simulink library "Lib_FileLoggerMultipacket"  (R2012b)
settings: Solver=ode45  StartTime=0.0  StopTime=10.0  RelTol=1e-3
undefined symbols (not defined in the file): macaddr, modelConstants
libraries: Lib_FileLoggerMultipacket x5, simulink x3, xpcutilitieslib x1, dspswit3 x1, dspmtrx3 x1, libBusSerialize x1
settings Model: Creator=gilja  LastModifiedBy=Chethan

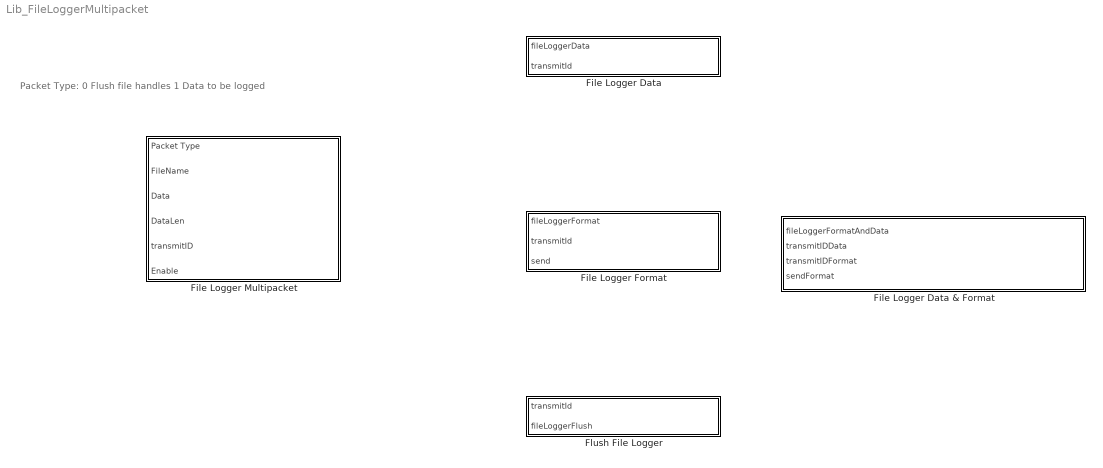
== system Lib_FileLoggerMultipacket ==
  note: Packet Type:
      | 0 Flush file handles
      | 1 Data to be logged
  File Logger Data : Subsystem
  File Logger Data & Format : Subsystem
  File Logger Format : Subsystem
  File Logger Multipacket : Subsystem
  Flush File Logger : Subsystem

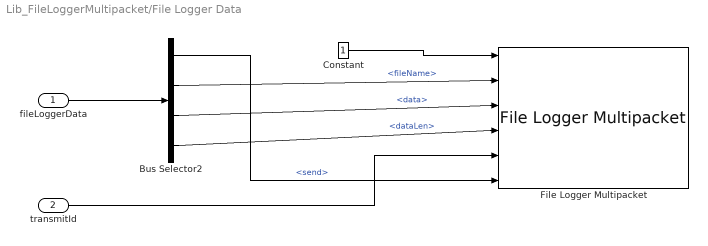
== system Lib_FileLoggerMultipacket/File Logger Data ==
  fileLoggerData : Inport  OutDataTypeStr=Bus: fileLoggerData
  transmitId : Inport  Port=2  OutDataTypeStr=uint8
  Bus Selector2 : BusSelector  OutputSignals=send,fileName,data,dataLen
  Constant : Constant  OutDataTypeStr=boolean
  File Logger Multipacket : Lib_FileLoggerMultipacket/File Logger Multipacket
  wires:
  fileLoggerData/1 -> Bus Selector2/1
  Constant/1 -> File Logger Multipacket/1
  Bus Selector2/1 -> File Logger Multipacket/6  "<send>"
  Bus Selector2/4 -> File Logger Multipacket/4  "<dataLen>"
  Bus Selector2/3 -> File Logger Multipacket/3  "<data>"
  Bus Selector2/2 -> File Logger Multipacket/2  "<fileName>"
  transmitId/1 -> File Logger Multipacket/5

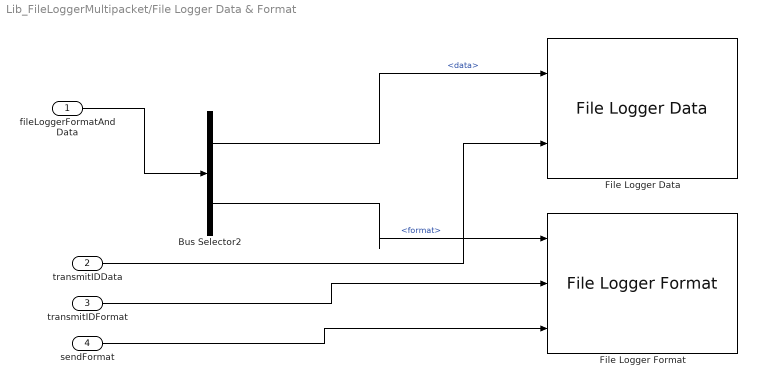
== system Lib_FileLoggerMultipacket/File Logger Data & Format ==
  fileLoggerFormatAndData : Inport  OutDataTypeStr=Bus: fileLoggerFormatAndData
  transmitIDData : Inport  Port=2  OutDataTypeStr=uint8
  transmitIDFormat : Inport  Port=3  OutDataTypeStr=uint8
  sendFormat : Inport  Port=4  OutDataTypeStr=boolean
  Bus Selector2 : BusSelector  OutputSignals=data,format
  File Logger Data : Lib_FileLoggerMultipacket/File Logger Data
  File Logger Format : Lib_FileLoggerMultipacket/File Logger Format
  wires:
  fileLoggerFormatAndData/1 -> Bus Selector2/1
  Bus Selector2/1 -> File Logger Data/1  "<data>"
  Bus Selector2/2 -> File Logger Format/1  "<format>"
  sendFormat/1 -> File Logger Format/3
  transmitIDData/1 -> File Logger Data/2
  transmitIDFormat/1 -> File Logger Format/2

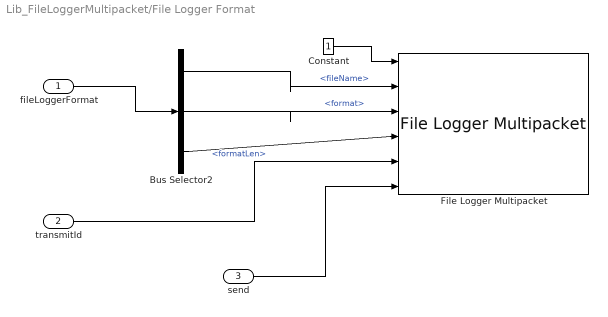
== system Lib_FileLoggerMultipacket/File Logger Format ==
  fileLoggerFormat : Inport  OutDataTypeStr=Bus: fileLoggerFormat
  transmitId : Inport  Port=2  OutDataTypeStr=uint8
  send : Inport  Port=3  OutDataTypeStr=boolean
  Bus Selector2 : BusSelector  OutputSignals=fileName,format,formatLen
  Constant : Constant  OutDataTypeStr=boolean
  File Logger Multipacket : Lib_FileLoggerMultipacket/File Logger Multipacket
  wires:
  fileLoggerFormat/1 -> Bus Selector2/1
  Constant/1 -> File Logger Multipacket/1
  Bus Selector2/3 -> File Logger Multipacket/4  "<formatLen>"
  Bus Selector2/2 -> File Logger Multipacket/3  "<format>"
  Bus Selector2/1 -> File Logger Multipacket/2  "<fileName>"
  send/1 -> File Logger Multipacket/6
  transmitId/1 -> File Logger Multipacket/5

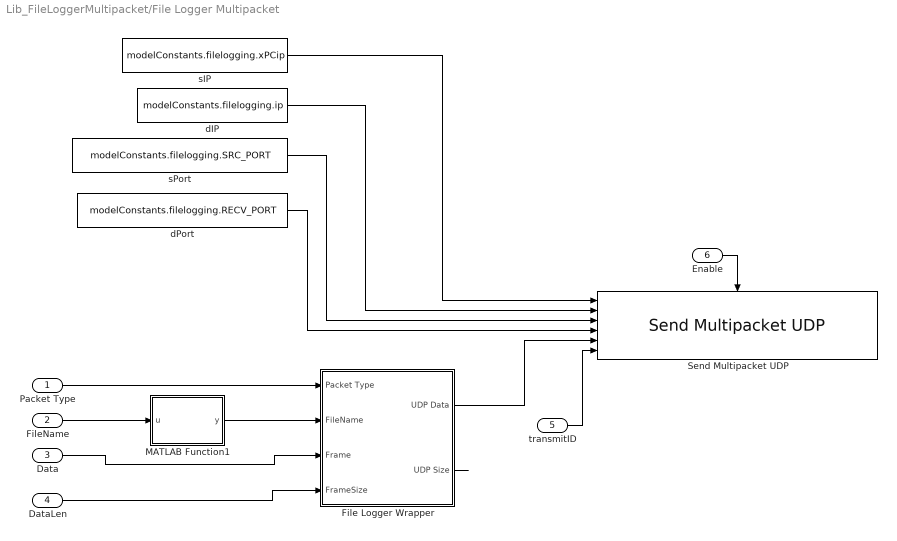
== system Lib_FileLoggerMultipacket/File Logger Multipacket ==
  Packet Type : Inport
  FileName : Inport  Port=2
  Data : Inport  Port=3
  DataLen : Inport  Port=4
  transmitID : Inport  Port=5
  Enable : Inport  Port=6
  File Logger Wrapper : Subsystem
  MATLAB Function1 : MATLAB Function  TreatAsAtomicUnit=on
  Send Multipacket UDP : libBusSerialize/Send Multipacket UDP  destMac=macaddr('ff:ff:ff:ff:ff:ff')  ID=2  prependHeader=off
  dIP : Constant  Value=modelConstants.filelogging.ip  OutDataTypeStr=uint8
  dPort : Constant  Value=modelConstants.filelogging.RECV_PORT  OutDataTypeStr=uint16
  sIP : Constant  Value=modelConstants.filelogging.xPCip  OutDataTypeStr=uint8
  sPort : Constant  Value=modelConstants.filelogging.SRC_PORT  OutDataTypeStr=uint16
  wires:
  FileName/1 -> MATLAB Function1/1(u)
  Packet Type/1 -> File Logger Wrapper/1(Packet Type)
  MATLAB Function1/1(y) -> File Logger Wrapper/2(FileName)
  File Logger Wrapper/2(UDP Size) -> ?
  DataLen/1 -> File Logger Wrapper/4(FrameSize)
  Data/1 -> File Logger Wrapper/3(Frame)
  Enable/1 -> Send Multipacket UDP/Enable
  dPort/1 -> Send Multipacket UDP/4
  sPort/1 -> Send Multipacket UDP/3
  dIP/1 -> Send Multipacket UDP/2
  sIP/1 -> Send Multipacket UDP/1
  File Logger Wrapper/1(UDP Data) -> Send Multipacket UDP/5
  transmitID/1 -> Send Multipacket UDP/6

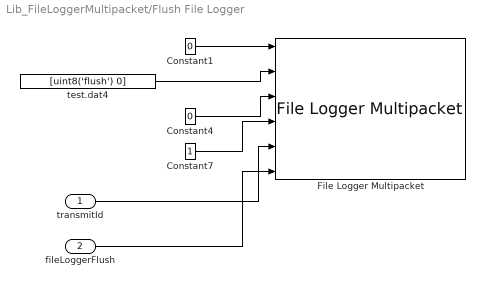
== system Lib_FileLoggerMultipacket/Flush File Logger ==
  transmitId : Inport  OutDataTypeStr=uint8
  fileLoggerFlush : Inport  Port=2  OutDataTypeStr=boolean
  Constant1 : Constant  Value=0  OutDataTypeStr=boolean
  Constant4 : Constant  Value=0  OutDataTypeStr=uint8
  Constant7 : Constant  OutDataTypeStr=uint16
  File Logger Multipacket : Lib_FileLoggerMultipacket/File Logger Multipacket
  test.dat4 : Constant  Value=[uint8('flush') 0]  OutDataTypeStr=uint8
  wires:
  Constant4/1 -> File Logger Multipacket/3
  fileLoggerFlush/1 -> File Logger Multipacket/6
  Constant7/1 -> File Logger Multipacket/4
  Constant1/1 -> File Logger Multipacket/1
  test.dat4/1 -> File Logger Multipacket/2
  transmitId/1 -> File Logger Multipacket/5

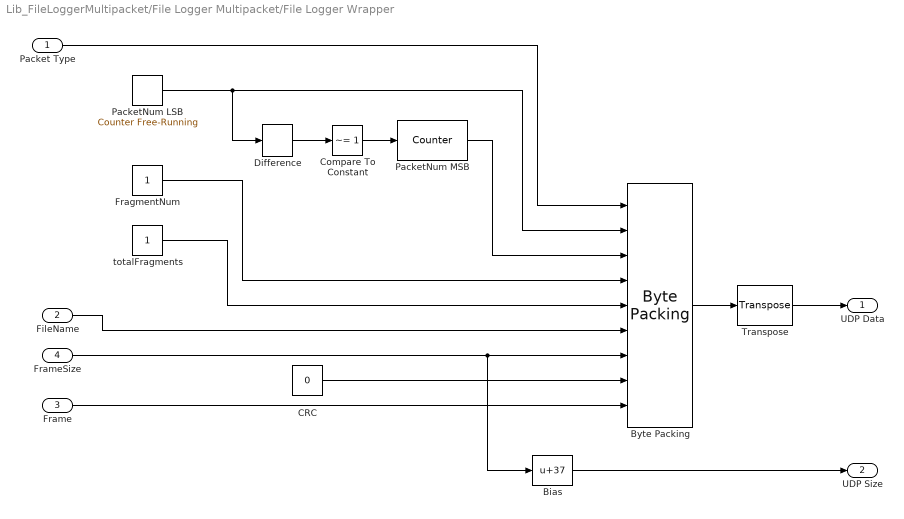
== system Lib_FileLoggerMultipacket/File Logger Multipacket/File Logger Wrapper ==
  Packet Type : Inport
  FileName : Inport  Port=2
  Frame : Inport  Port=3
  FrameSize : Inport  Port=4
  Bias : Bias  Bias=37
  "Byte Packing " : xpcutilitieslib/Byte Packing   MaskPackedDataType=uint8  MaskUnpackedDataTypes={'boolean' 'uint32' 'uint32' 'uint8' 'uint8' 'uint8' 'uint16' 'uint32' 'uint8'}  MaskAlignment=1
  CRC : Constant  Value=0  OutDataTypeStr=uint32
  Compare To Constant : simulink/Logic and Bit Operations/Compare To Constant  relop=~=  const=1  OutDataTypeStr=uint8  ZeroCross=off
  Difference : simulink/Discrete/Difference  ICPrevInput=0  InputProcessing=Inherited  OutMin=[]  OutMax=[]  OutDataType=fixdt(1, 16)  OutScaling=2^-10  DoSatur=off
  FragmentNum : Constant  OutDataTypeStr=uint8
  PacketNum LSB : simulink/Sources/Counter Free-Running  NumBits=32  tsamp=-1
  PacketNum MSB : dspswit3/Counter  Direction=Up  CountEvent=Non-zero sample  CounterSize=32 bits  MaxCount=255  InitialCount=0  Output=Count  HitValue=32  ResetInput=off  SamplesPerFrame=1  Ts=1  CntDtype=uint32  HitDtype=Logical
  Transpose : dspmtrx3/Transpose  Hermitian=off  overflowFlag=off
  totalFragments : Constant  OutDataTypeStr=uint8
  UDP Data : Outport
  UDP Size : Outport  Port=2
  wires:
  Transpose/1 -> UDP Data/1
  "Byte Packing "/1 -> Transpose/1
  Frame/1 -> "Byte Packing "/9
  FrameSize/1 -> Bias/1, "Byte Packing "/7
  CRC/1 -> "Byte Packing "/8
  PacketNum MSB/1 -> "Byte Packing "/3
  Compare To Constant/1 -> PacketNum MSB/1
  Difference/1 -> Compare To Constant/1
  Packet Type/1 -> "Byte Packing "/1
  PacketNum LSB/1 -> "Byte Packing "/2, Difference/1
  FragmentNum/1 -> "Byte Packing "/4
  totalFragments/1 -> "Byte Packing "/5
  FileName/1 -> "Byte Packing "/6
  Bias/1 -> UDP Size/1

== matlab function Lib_FileLoggerMultipacket/File Logger Multipacket/MATLAB Function1 ==
  data: u input; y output
function y = padFileName(u)

z = uint8(zeros(20, 1));

z(1:length(u)) = u;

y = z';
